simulink model "wind_turbine"  (Simulink 7.8)
settings: Solver=ode45  StartTime=0.0  StopTime=inf  RelTol=1e-3
values from neighbouring files (symbols this model uses):
  q = [x2;y2;c2;x3;y3;z3;a3;b3;c3;x4;y4;z4;b4;c4;x5;y5;z5;b5;c5;a6;b6;c6;a7;xSun;ySun;zSun;bSun;cSun;xPla1;yPla1;zPla1;bPla1;cPla1;xPla2;yPla2;zPla2;bPla2;cPla2;xPla3;yPla3;zPla3;bPla3;cPla3;xSecSt;ySecSt;zSecSt;bSecSt;cSecSt;a4;a5;aSun;aPla1;aPla2;aPla3;aSecSt;]    [environment.m]
settings Model: Creator=imac  LastModifiedBy=aitor
settings DebuggingCC: FcnCallInpInsideContextMsg=Use local settings

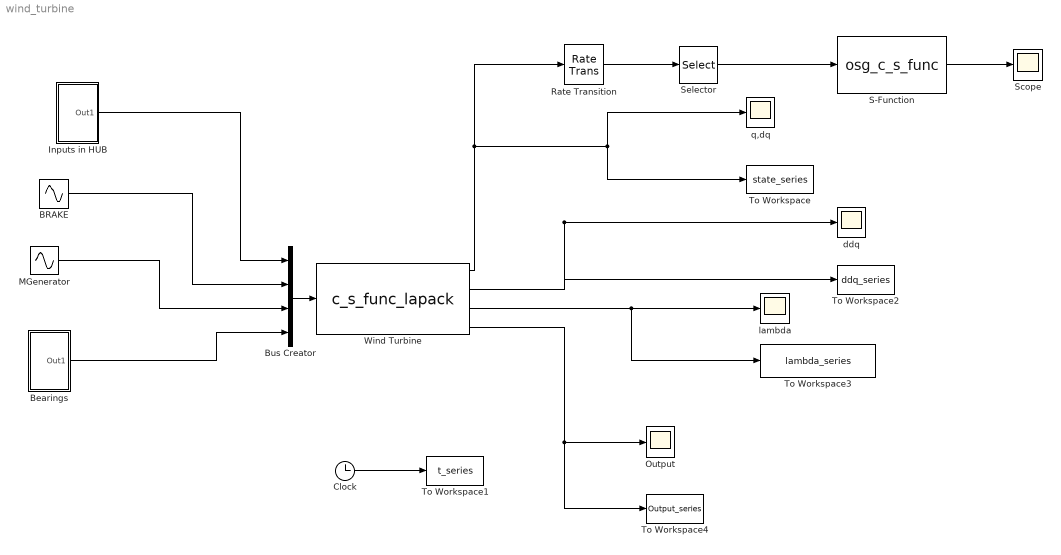
== system wind_turbine ==
  BRAKE : Sin  Amplitude=0  Frequency=0  Phase=pi/2  SampleTime=0
  Bearings : Subsystem
  Bus Creator : BusCreator
  Clock : Clock
  Inputs in HUB : Subsystem
  MGenerator : Sin  Amplitude=0  Frequency=0  Phase=pi/2  SampleTime=0
  Output : Scope
      settings: YMin=0  YMax=1300  SaveName=ScopeData3  SampleInput=on  SampleTime=0.01
  Rate Transition : RateTransition  OutPortSampleTime=0.04
  S-Function : S-Function  FunctionName=osg_c_s_func  EnableBusSupport=off
  Scope : Scope
      settings: SaveName=ScopeData4
  Selector : Selector  InputPortWidth=2*length(q)  IndexOptions=Index vector (dialog)  Indices=1:1:length(q)  OutputSizes=1
  To Workspace : ToWorkspace  VariableName=state_series  SampleTime=0.01  SaveFormat=Array
  To Workspace1 : ToWorkspace  VariableName=t_series  SampleTime=0.01  SaveFormat=Array
  To Workspace2 : ToWorkspace  VariableName=ddq_series  SampleTime=0.01  SaveFormat=Array
  To Workspace3 : ToWorkspace  VariableName=lambda_series  SampleTime=0.01  SaveFormat=Array
  To Workspace4 : ToWorkspace  VariableName=Output_series  SampleTime=0.01  SaveFormat=Array
  Wind Turbine : S-Function  FunctionName=c_s_func_lapack  Parameters=q dq param  EnableBusSupport=off
      mask Type: S-function: mycsfunc
      mask Description: This is a S-function that does the continuous state space system.
      mask Display: disp('[M , Phi_q''] [ddq]\n[Phi_q , 0] [lambda]\n=\n [Q ] \n   [gamma] ');
  ddq : Scope
      settings: YMin=-500  YMax=300  SampleInput=on  SampleTime=0.01
  lambda : Scope
      settings: YMin=-1750  YMax=1000  SaveName=ScopeData2  SampleInput=on  SampleTime=0.01
  q,dq : Scope
      settings: YMin=-0.035  YMax=0.045  SampleInput=on  SampleTime=0.01
  wires:
  Clock/1 -> To Workspace1/1
  Wind Turbine/1 -> q,dq/1, To Workspace/1, Rate Transition/1
  Wind Turbine/2 -> ddq/1, To Workspace2/1
  Wind Turbine/3 -> lambda/1, To Workspace3/1
  Wind Turbine/4 -> Output/1, To Workspace4/1
  Selector/1 -> S-Function/1
  S-Function/1 -> Scope/1
  Inputs in HUB/1(Out1) -> Bus Creator/1
  Bus Creator/1 -> Wind Turbine/1
  BRAKE/1 -> Bus Creator/2
  MGenerator/1 -> Bus Creator/3
  Bearings/1(Out1) -> Bus Creator/4
  Rate Transition/1 -> Selector/1

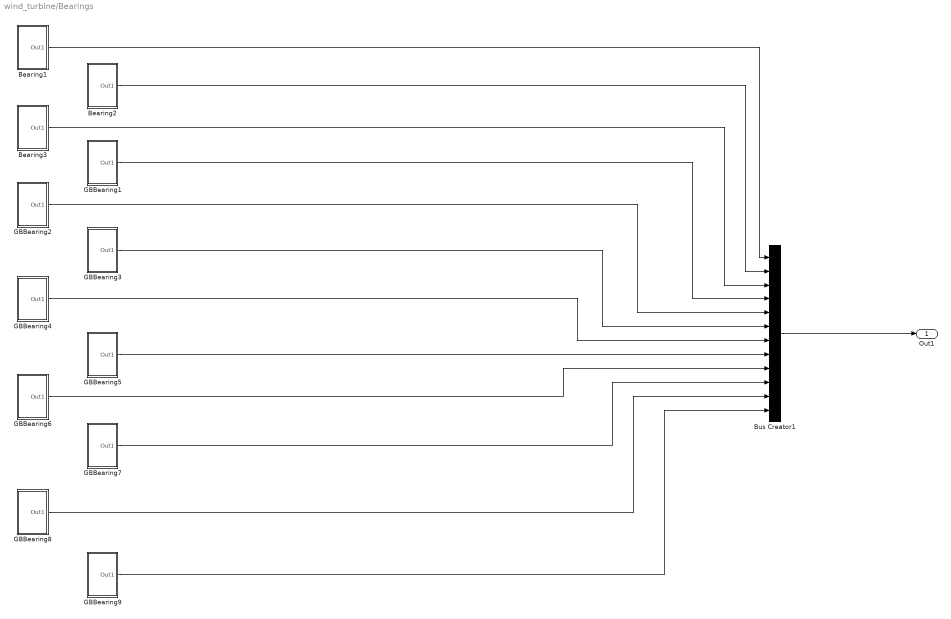
== system wind_turbine/Bearings ==
  " GBBearing2" : Subsystem
  Bearing1 : Subsystem
  Bearing2 : Subsystem
  Bearing3 : Subsystem
  Bus Creator1 : BusCreator  Inputs=12
  GBBearing1 : Subsystem
  GBBearing3 : Subsystem
  GBBearing4 : Subsystem
  GBBearing5 : Subsystem
  GBBearing6 : Subsystem
  GBBearing7 : Subsystem
  GBBearing8 : Subsystem
  GBBearing9 : Subsystem
  Out1 : Outport
  wires:
  Bearing1/1(Out1) -> Bus Creator1/1
  Bearing2/1(Out1) -> Bus Creator1/2
  Bearing3/1(Out1) -> Bus Creator1/3
  GBBearing1/1(Out1) -> Bus Creator1/4
  Bus Creator1/1 -> Out1/1
  " GBBearing2"/1(Out1) -> Bus Creator1/5
  GBBearing3/1(Out1) -> Bus Creator1/6
  GBBearing4/1(Out1) -> Bus Creator1/7
  GBBearing5/1(Out1) -> Bus Creator1/8
  GBBearing6/1(Out1) -> Bus Creator1/9
  GBBearing7/1(Out1) -> Bus Creator1/10
  GBBearing8/1(Out1) -> Bus Creator1/11
  GBBearing9/1(Out1) -> Bus Creator1/12

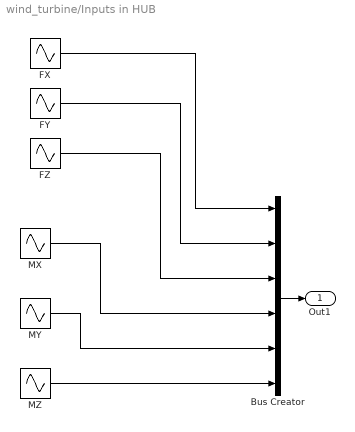
== system wind_turbine/Inputs in HUB ==
  Bus Creator : BusCreator  Inputs=6
  FX : Sin  Description=FX  Amplitude=0  Frequency=0  Phase=pi/2  SampleTime=0
  FY : Sin  Amplitude=0  Frequency=0  Phase=pi/2  SampleTime=0
  FZ : Sin  Amplitude=0  Frequency=0  Phase=pi/2  SampleTime=0
  MX : Sin  Amplitude=0  Frequency=0  Phase=pi/2  SampleTime=0
  MY : Sin  Amplitude=0  Frequency=0  Phase=pi/2  SampleTime=0
  MZ : Sin  Amplitude=0  Frequency=0  Phase=pi/2  SampleTime=0
  Out1 : Outport
  wires:
  FX/1 -> Bus Creator/1
  FY/1 -> Bus Creator/2
  MX/1 -> Bus Creator/4
  MY/1 -> Bus Creator/5
  MZ/1 -> Bus Creator/6
  FZ/1 -> Bus Creator/3
  Bus Creator/1 -> Out1/1

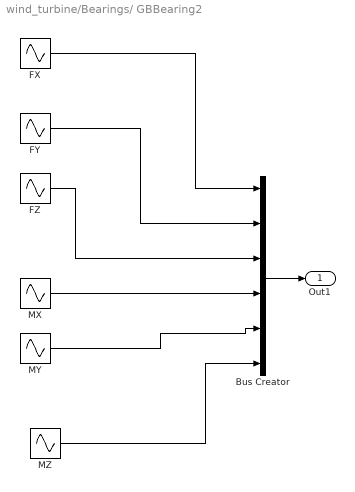
== system wind_turbine/Bearings/ GBBearing2 ==
  Bus Creator : BusCreator  Inputs=6
  FX : Sin  Description=FX  Amplitude=0  Frequency=0  Phase=pi/2  SampleTime=0
  FY : Sin  Amplitude=0  Frequency=0  Phase=pi/2  SampleTime=0
  FZ : Sin  Amplitude=0  Frequency=0  Phase=pi/2  SampleTime=0
  MX : Sin  Amplitude=0  Frequency=0  Phase=pi/2  SampleTime=0
  MY : Sin  Amplitude=0  Frequency=0  Phase=pi/2  SampleTime=0
  MZ : Sin  Amplitude=0  Frequency=0  Phase=pi/2  SampleTime=0
  Out1 : Outport
  wires:
  FX/1 -> Bus Creator/1
  FY/1 -> Bus Creator/2
  MX/1 -> Bus Creator/4
  MY/1 -> Bus Creator/5
  MZ/1 -> Bus Creator/6
  FZ/1 -> Bus Creator/3
  Bus Creator/1 -> Out1/1

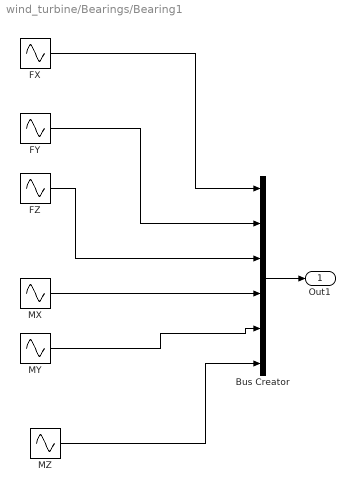
== system wind_turbine/Bearings/Bearing1 ==
  Bus Creator : BusCreator  Inputs=6
  FX : Sin  Description=FX  Amplitude=0  Frequency=0  Phase=pi/2  SampleTime=0
  FY : Sin  Amplitude=0  Frequency=0  Phase=pi/2  SampleTime=0
  FZ : Sin  Amplitude=0  Frequency=0  Phase=pi/2  SampleTime=0
  MX : Sin  Amplitude=0  Frequency=0  Phase=pi/2  SampleTime=0
  MY : Sin  Amplitude=0  Frequency=0  Phase=pi/2  SampleTime=0
  MZ : Sin  Amplitude=0  Frequency=0  Phase=pi/2  SampleTime=0
  Out1 : Outport
  wires:
  FX/1 -> Bus Creator/1
  FY/1 -> Bus Creator/2
  MX/1 -> Bus Creator/4
  MY/1 -> Bus Creator/5
  MZ/1 -> Bus Creator/6
  FZ/1 -> Bus Creator/3
  Bus Creator/1 -> Out1/1

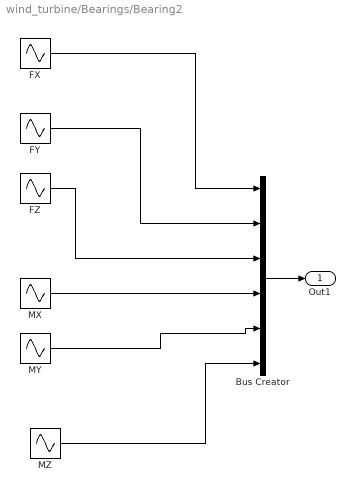
== system wind_turbine/Bearings/Bearing2 ==
  Bus Creator : BusCreator  Inputs=6
  FX : Sin  Description=FX  Amplitude=0  Frequency=0  Phase=pi/2  SampleTime=0
  FY : Sin  Amplitude=0  Frequency=0  Phase=pi/2  SampleTime=0
  FZ : Sin  Amplitude=0  Frequency=pi/2  SampleTime=0
  MX : Sin  Amplitude=0  Frequency=0  Phase=pi/2  SampleTime=0
  MY : Sin  Amplitude=0  Frequency=0  Phase=pi/2  SampleTime=0
  MZ : Sin  Amplitude=0  Frequency=0  Phase=pi/2  SampleTime=0
  Out1 : Outport
  wires:
  FX/1 -> Bus Creator/1
  FY/1 -> Bus Creator/2
  MX/1 -> Bus Creator/4
  MY/1 -> Bus Creator/5
  MZ/1 -> Bus Creator/6
  FZ/1 -> Bus Creator/3
  Bus Creator/1 -> Out1/1

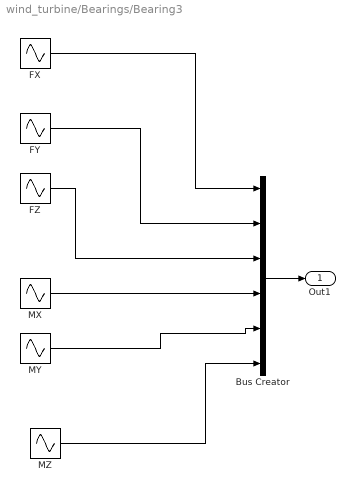
== system wind_turbine/Bearings/Bearing3 ==
  Bus Creator : BusCreator  Inputs=6
  FX : Sin  Description=FX  Amplitude=0  Frequency=0  Phase=pi/2  SampleTime=0
  FY : Sin  Amplitude=0  Frequency=0  Phase=pi/2  SampleTime=0
  FZ : Sin  Amplitude=0  Frequency=0  Phase=pi/2  SampleTime=0
  MX : Sin  Amplitude=0  Frequency=0  Phase=pi/2  SampleTime=0
  MY : Sin  Amplitude=0  Frequency=0  Phase=pi/2  SampleTime=0
  MZ : Sin  Amplitude=0  Frequency=0  Phase=pi/2  SampleTime=0
  Out1 : Outport
  wires:
  FX/1 -> Bus Creator/1
  FY/1 -> Bus Creator/2
  MX/1 -> Bus Creator/4
  MY/1 -> Bus Creator/5
  MZ/1 -> Bus Creator/6
  FZ/1 -> Bus Creator/3
  Bus Creator/1 -> Out1/1

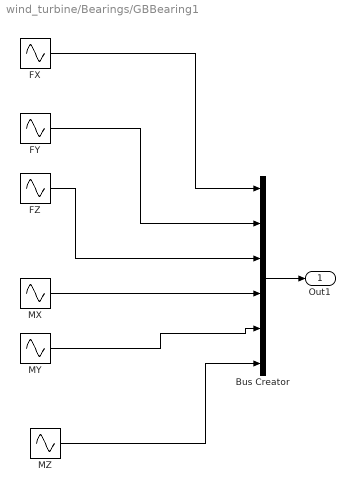
== system wind_turbine/Bearings/GBBearing1 ==
  Bus Creator : BusCreator  Inputs=6
  FX : Sin  Description=FX  Amplitude=0  Frequency=0  Phase=pi/2  SampleTime=0
  FY : Sin  Amplitude=0  Frequency=0  Phase=pi/2  SampleTime=0
  FZ : Sin  Amplitude=0  Frequency=pi/2  SampleTime=0
  MX : Sin  Amplitude=0  Frequency=0  Phase=pi/2  SampleTime=0
  MY : Sin  Amplitude=0  Frequency=0  Phase=pi/2  SampleTime=0
  MZ : Sin  Amplitude=0  Frequency=0  Phase=pi/2  SampleTime=0
  Out1 : Outport
  wires:
  FX/1 -> Bus Creator/1
  FY/1 -> Bus Creator/2
  MX/1 -> Bus Creator/4
  MY/1 -> Bus Creator/5
  MZ/1 -> Bus Creator/6
  FZ/1 -> Bus Creator/3
  Bus Creator/1 -> Out1/1

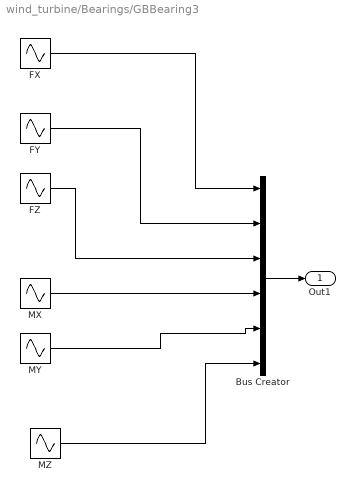
== system wind_turbine/Bearings/GBBearing3 ==
  Bus Creator : BusCreator  Inputs=6
  FX : Sin  Description=FX  Amplitude=0  Frequency=0  Phase=pi/2  SampleTime=0
  FY : Sin  Amplitude=0  Frequency=0  Phase=pi/2  SampleTime=0
  FZ : Sin  Amplitude=0  Frequency=0  Phase=pi/2  SampleTime=0
  MX : Sin  Amplitude=0  Frequency=0  Phase=pi/2  SampleTime=0
  MY : Sin  Amplitude=0  Frequency=0  Phase=pi/2  SampleTime=0
  MZ : Sin  Amplitude=0  Frequency=0  Phase=pi/2  SampleTime=0
  Out1 : Outport
  wires:
  FX/1 -> Bus Creator/1
  FY/1 -> Bus Creator/2
  MX/1 -> Bus Creator/4
  MY/1 -> Bus Creator/5
  MZ/1 -> Bus Creator/6
  FZ/1 -> Bus Creator/3
  Bus Creator/1 -> Out1/1

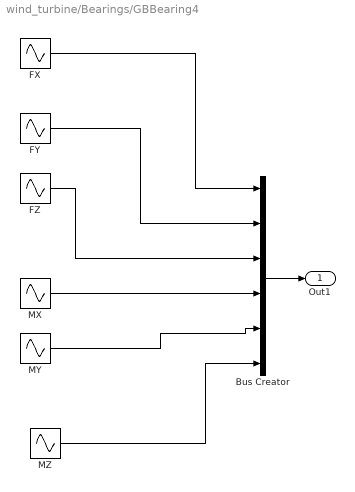
== system wind_turbine/Bearings/GBBearing4 ==
  Bus Creator : BusCreator  Inputs=6
  FX : Sin  Description=FX  Amplitude=0  Frequency=0  Phase=pi/2  SampleTime=0
  FY : Sin  Amplitude=0  Frequency=0  Phase=pi/2  SampleTime=0
  FZ : Sin  Amplitude=0  Frequency=0  Phase=pi/2  SampleTime=0
  MX : Sin  Amplitude=0  Frequency=0  Phase=pi/2  SampleTime=0
  MY : Sin  Amplitude=0  Frequency=0  Phase=pi/2  SampleTime=0
  MZ : Sin  Amplitude=0  Frequency=0  Phase=pi/2  SampleTime=0
  Out1 : Outport
  wires:
  FX/1 -> Bus Creator/1
  FY/1 -> Bus Creator/2
  MX/1 -> Bus Creator/4
  MY/1 -> Bus Creator/5
  MZ/1 -> Bus Creator/6
  FZ/1 -> Bus Creator/3
  Bus Creator/1 -> Out1/1

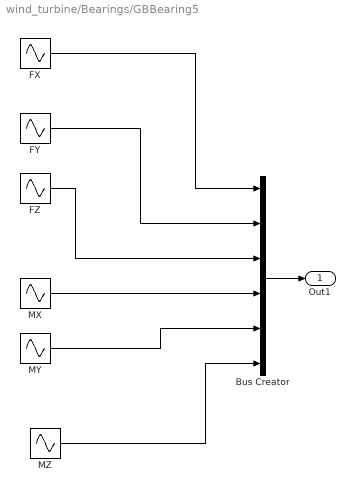
== system wind_turbine/Bearings/GBBearing5 ==
  Bus Creator : BusCreator  Inputs=6
  FX : Sin  Description=FX  Amplitude=0  Frequency=0  Phase=pi/2  SampleTime=0
  FY : Sin  Amplitude=0  Frequency=0  Phase=pi/2  SampleTime=0
  FZ : Sin  Amplitude=0  Frequency=0  Phase=pi/2  SampleTime=0
  MX : Sin  Amplitude=0  Frequency=0  Phase=pi/2  SampleTime=0
  MY : Sin  Amplitude=0  Frequency=0  Phase=pi/2  SampleTime=0
  MZ : Sin  Amplitude=0  Frequency=0  Phase=pi/2  SampleTime=0
  Out1 : Outport
  wires:
  FX/1 -> Bus Creator/1
  FY/1 -> Bus Creator/2
  MX/1 -> Bus Creator/4
  MY/1 -> Bus Creator/5
  MZ/1 -> Bus Creator/6
  FZ/1 -> Bus Creator/3
  Bus Creator/1 -> Out1/1

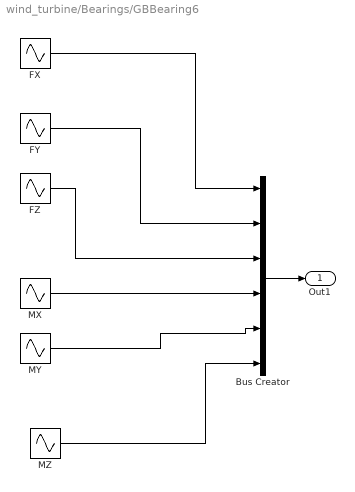
== system wind_turbine/Bearings/GBBearing6 ==
  Bus Creator : BusCreator  Inputs=6
  FX : Sin  Description=FX  Amplitude=0  Frequency=0  Phase=pi/2  SampleTime=0
  FY : Sin  Amplitude=0  Frequency=0  Phase=pi/2  SampleTime=0
  FZ : Sin  Amplitude=0  Frequency=0  Phase=pi/2  SampleTime=0
  MX : Sin  Amplitude=0  Frequency=0  Phase=pi/2  SampleTime=0
  MY : Sin  Amplitude=0  Frequency=0  Phase=pi/2  SampleTime=0
  MZ : Sin  Amplitude=0  Frequency=0  Phase=pi/2  SampleTime=0
  Out1 : Outport
  wires:
  FX/1 -> Bus Creator/1
  FY/1 -> Bus Creator/2
  MX/1 -> Bus Creator/4
  MY/1 -> Bus Creator/5
  MZ/1 -> Bus Creator/6
  FZ/1 -> Bus Creator/3
  Bus Creator/1 -> Out1/1

== system wind_turbine/Bearings/GBBearing7 ==
  Bus Creator : BusCreator  Inputs=6
  FX : Sin  Description=FX  Amplitude=0  Frequency=0  Phase=pi/2  SampleTime=0
  FY : Sin  Amplitude=0  Frequency=0  Phase=pi/2  SampleTime=0
  FZ : Sin  Amplitude=0  Frequency=100  Phase=pi/2  SampleTime=0
  MX : Sin  Amplitude=0  Frequency=0  Phase=pi/2  SampleTime=0
  MY : Sin  Amplitude=0  Frequency=0  Phase=pi/2  SampleTime=0
  MZ : Sin  Amplitude=0  Frequency=0  Phase=pi/2  SampleTime=0
  Out1 : Outport
  wires:
  FX/1 -> Bus Creator/1
  FY/1 -> Bus Creator/2
  MX/1 -> Bus Creator/4
  MY/1 -> Bus Creator/5
  MZ/1 -> Bus Creator/6
  FZ/1 -> Bus Creator/3
  Bus Creator/1 -> Out1/1

== system wind_turbine/Bearings/GBBearing8 ==
  Bus Creator : BusCreator  Inputs=6
  FX : Sin  Description=FX  Amplitude=0  Frequency=0  Phase=pi/2  SampleTime=0
  FY : Sin  Amplitude=0  Frequency=0  Phase=pi/2  SampleTime=0
  FZ : Sin  Amplitude=0  Frequency=100  Phase=pi/2  SampleTime=0
  MX : Sin  Amplitude=0  Frequency=0  Phase=pi/2  SampleTime=0
  MY : Sin  Amplitude=0  Frequency=0  Phase=pi/2  SampleTime=0
  MZ : Sin  Amplitude=0  Frequency=0  Phase=pi/2  SampleTime=0
  Out1 : Outport
  wires:
  FX/1 -> Bus Creator/1
  FY/1 -> Bus Creator/2
  MX/1 -> Bus Creator/4
  MY/1 -> Bus Creator/5
  MZ/1 -> Bus Creator/6
  FZ/1 -> Bus Creator/3
  Bus Creator/1 -> Out1/1

== system wind_turbine/Bearings/GBBearing9 ==
  Bus Creator : BusCreator  Inputs=6
  FX : Sin  Description=FX  Amplitude=0  Frequency=0  Phase=pi/2  SampleTime=0
  FY : Sin  Amplitude=0  Frequency=0  Phase=pi/2  SampleTime=0
  FZ : Sin  Amplitude=0  Frequency=0  Phase=pi/2  SampleTime=0
  MX : Sin  Amplitude=0  Frequency=0  Phase=pi/2  SampleTime=0
  MY : Sin  Amplitude=0  Frequency=0  Phase=pi/2  SampleTime=0
  MZ : Sin  Amplitude=0  Frequency=0  Phase=pi/2  SampleTime=0
  Out1 : Outport
  wires:
  FX/1 -> Bus Creator/1
  FY/1 -> Bus Creator/2
  MX/1 -> Bus Creator/4
  MY/1 -> Bus Creator/5
  MZ/1 -> Bus Creator/6
  FZ/1 -> Bus Creator/3
  Bus Creator/1 -> Out1/1
